simulink model "hydraulic_model"  (R2024a)
settings: Solver=ode23t  StartTime=0.0  StopTime=tEnd  FixedStep=1e-4  MaxStep=maxStep  RelTol=1e-2  AbsTol=1e-2
values from neighbouring files (symbols this model uses):
  boomHEArea = pi * (boomBoreDiameter/2)^2    (= 3117.24531052)    [init_model.m]
  boomREArea = pi * (boomBoreDiameter/2)^2 - pi*(boomRodDiameter/2)^2    (= 2410.38696347)    [init_model.m]
  swingDisplacement = 23.6    [init_model.m]
undefined symbols (not defined in the file or in its folder): ArmC, ArmR, AToTOrificeVector, BiPOrificeVector, BoomC, BoomR, boomValve, BToTOrificeVector, BucketC, BucketR, bucketValve, fluids, PToAOrificeVector, PToBOrificeVector, stickValve, SwingC, SwingR, swingValve, X, Y, Z
libraries: fl_lib x81, SimscapeFluids_lib x54, sm_lib x34, nesl_utility x29, spsFirstOrderFilterLib x4
(part 1 of 5)
settings Model: SimulationMode=accelerator  Creator=The MathWorks, Inc.  LastModifiedBy=jommsy
settings SolverCC: MaxConsecutiveMinStep=10  ZeroCrossAlgorithm=Adaptive  AlgebraicLoopSolver=TrustRegion  DecoupledContinuousIntegration=on  MinimalZcImpactIntegration=on
settings DataIOCC: SaveOutput=off  DSMLogging=off  OutputTimes=[0:0.02:20]
settings OptimizationCC: UseDivisionForNetSlopeComputation=UseDivisionForReciprocalsOfIntegersOnly  StateBitsets=on  DataBitsets=on
settings DebuggingCC: IgnoredZcDiagnostic=none  IntegerOverflowMsg=error  UnconnectedInputMsg=warning  UnconnectedOutputMsg=warning  UnconnectedLineMsg=warning  ArithmeticOperatorsInVariantConditions=warning
settings ModelReferenceCC: EnableRefExpFcnMdlSchedulingChecks=on
settings SFSimCC: MATLABDynamicMemAlloc=off  CustomCodeUndefinedFunction=UseInterfaceOnly
settings RTWCC: GPUComputeCapability=3.5
settings GRTTargetCC: UtilityFuncGeneration=Shared location
settings ExplorerConfigSet: SimMechanicsOpenEditorOnUpdate=off

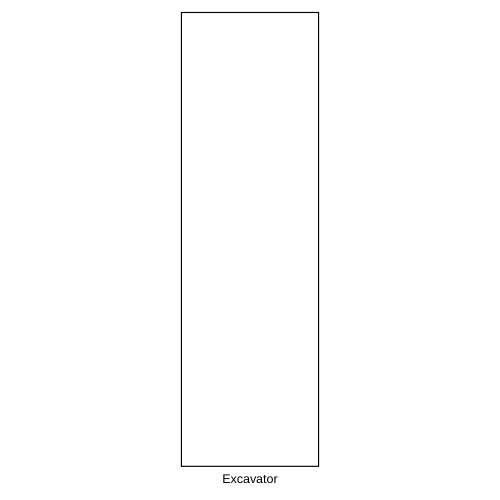
[thumbnail: Simulink's stored preview of the top-level diagram]
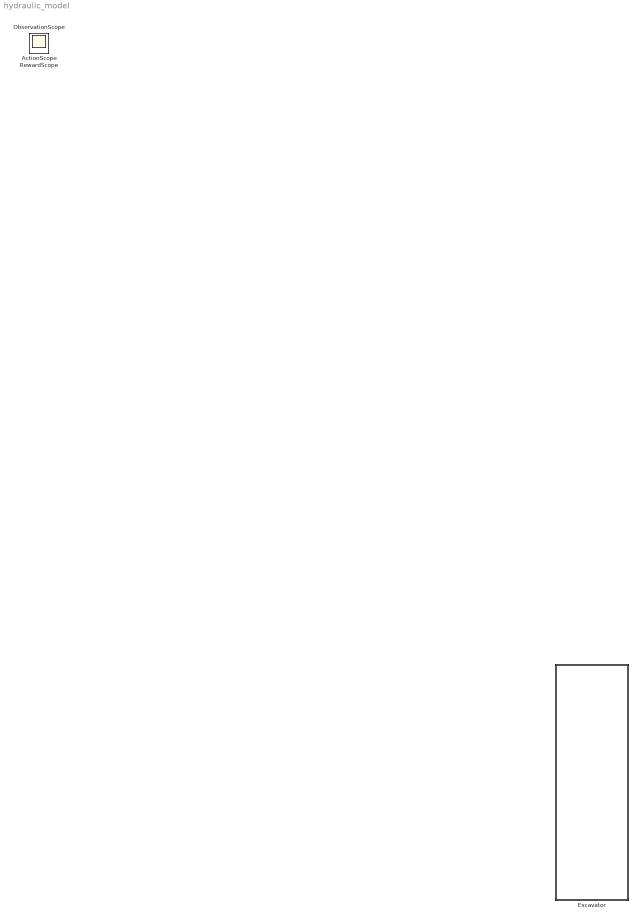
== system hydraulic_model ==
  Excavator : Subsystem
  ActionScope : Scope
  ObservationScope : Scope
  RewardScope : Scope

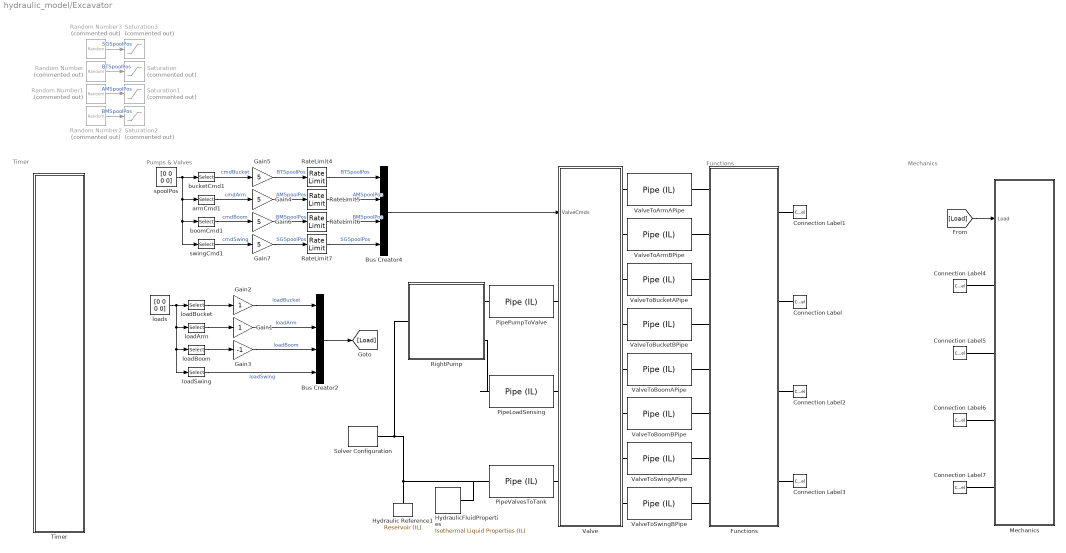
== system hydraulic_model/Excavator ==
  note: Functions
  note: Pumps & Valves
  note: Timer
  note: Mechanics
  Bus Creator2 : BusCreator  Inputs=4
  Bus Creator4 : BusCreator  Inputs=4
  Connection Label : ConnectionLabel  Label=ArmCyl
  Connection Label1 : ConnectionLabel  Label=BucketCyl
  Connection Label2 : ConnectionLabel  Label=BoomCyl
  Connection Label3 : ConnectionLabel  Label=SwingMotor
  Connection Label4 : ConnectionLabel  Label=ArmCyl
  Connection Label5 : ConnectionLabel  Label=BucketCyl
  Connection Label6 : ConnectionLabel  Label=BoomCyl
  Connection Label7 : ConnectionLabel  Label=SwingMotor
  Functions : Subsystem
      mask Display: image('Hydraulic_Actuators_All_IMAGE.png');
  Gain1 : Gain
  Gain2 : Gain
  Gain3 : Gain  Gain=-1
  Gain{4..7} (4 alike) : Gain  Gain=5
  Hydraulic Reference1 : fl_lib/Isothermal Liquid/Elements/Reservoir (IL)  reservoir_type=foundation.enum.constant_controlled.constant  pressure_spec=foundation.enum.pressure_spec.atmospheric  reservoir_pressure=0.101325 MPa
  HydraulicFluidProperties : fl_lib/Isothermal Liquid/Utilities/Isothermal Liquid Properties (IL)  rho_L_atm=870 kg/m^3  bulk_modulus_model=foundation.enum.bulk_modulus_model.const  beta_gain=6  beta_L_atm=1.45e9 Pa  nu_atm=46 mm^2/s  p_atm=0.101325 MPa  p_min=0.1 Pa  properties_range_check=simscape.enum.assert.action.error  air_fraction=0.005  polytropic_index=1.0  rho_g_atm=1.225 kg/m^3  air_dissolution_model=simscape.enum.onoff.off  p_crit=3 MPa
  Mechanics : Subsystem
      settings: PortSchema="{\"entries\":[{\"content\":{\"sides\":[{\"content\":{},\"type\":\"ConnectorPlacement.EquallySpacedRectSide\",\"uuid\":\"df542c6c-93e0-4cd8-a234-068f710ec41b\"},{\"content\":{\"side\":\"RIGHT\"},\"type\":\"ConnectorPlacement.EquallySpacedRectSide\",\"uuid\":\"8b36ef69-95bb-49de-9017-375655dff0aa\"},{\"content\":{\"connectorIds\":[\"In1\",\"LConn1\",\"LConn2\",\"LConn3\",\"LConn4\"],\"side\":\"TOP\"},\"type\":\"ConnectorPlacement.EquallySpacedRectSide\",\"uuid\":\"d3e749b5-c6b1-4a0f-a6f8-f63c6bfd6ba8\"}]},\"type\":\"ConnectorPlacement.EquallySpacedConnector\",\"uuid\":\"9d57a862-0266-4ba5-b197-b3f576208194\"}],\"packageUris\":[\"http://schema.mathworks.com/mf0/Connector/R2020b\"],\"version\":\"1.0\"}"
      mask Display: image('Excavator_Cylinder_CalcForce_IMAGE.png', [0,0,0,0,80,80]);
  PipeLoadSensing : fl_lib/Isothermal Liquid/Elements/Pipe (IL)  length=pipeLength mm  area=pipeCrossSectArea mm^2  Dh=pipeHydraulicDiam mm  length_add=1 m  roughness=15e-6 m  Re_lam=2000  Re_tur=4000  shape_factor=64  dynamic_compressibility=simscape.enum.onoff.off  inertia=simscape.enum.onoff.off  p0=0.101325 MPa  mdot0=0 kg/s
      settings: InternalSimscapePortConfiguration="{\"Bottom\":[],\"Left\":[{\"id\":\"A\",\"label\":\"A\",\"type\":\"foundation.isothermal_liquid.isothermal_liquid\"}],\"Right\":[{\"id\":\"B\",\"label\":\"B\",\"type\":\"foundation.isothermal_liquid.isothermal_liquid\"}],\"Top\":[]}"
  PipePumpToValve : fl_lib/Isothermal Liquid/Elements/Pipe (IL)  length=pipeLength mm  area=pipeCrossSectArea mm^2  Dh=pipeHydraulicDiam mm  length_add=1 m  roughness=15e-6 m  Re_lam=2000  Re_tur=4000  shape_factor=64  dynamic_compressibility=simscape.enum.onoff.off  inertia=simscape.enum.onoff.off  p0=0.101325 MPa  mdot0=0 kg/s
      settings: InternalSimscapePortConfiguration="{\"Bottom\":[],\"Left\":[{\"id\":\"A\",\"label\":\"A\",\"type\":\"foundation.isothermal_liquid.isothermal_liquid\"}],\"Right\":[{\"id\":\"B\",\"label\":\"B\",\"type\":\"foundation.isothermal_liquid.isothermal_liquid\"}],\"Top\":[]}"
  PipeValvesToTank : fl_lib/Isothermal Liquid/Elements/Pipe (IL)  length=pipeLength mm  area=pipeCrossSectArea mm^2  Dh=pipeHydraulicDiam mm  length_add=1 m  roughness=15e-6 m  Re_lam=2000  Re_tur=4000  shape_factor=64  dynamic_compressibility=simscape.enum.onoff.off  inertia=simscape.enum.onoff.off  p0=0.101325 MPa  mdot0=0 kg/s
      settings: InternalSimscapePortConfiguration="{\"Bottom\":[],\"Left\":[{\"id\":\"A\",\"label\":\"A\",\"type\":\"foundation.isothermal_liquid.isothermal_liquid\"}],\"Right\":[{\"id\":\"B\",\"label\":\"B\",\"type\":\"foundation.isothermal_liquid.isothermal_liquid\"}],\"Top\":[]}"
  Random Number : RandomNumber  Commented=on  Variance=0.3  SampleTime=0.02
  Random Number1 : RandomNumber  Commented=on  Variance=0.3  Seed=1000  SampleTime=0.02
  Random Number2 : RandomNumber  Commented=on  Variance=0.3  Seed=20  SampleTime=0.02
  Random Number3 : RandomNumber  Commented=on  Variance=0.3  Seed=800  SampleTime=0.02
  RateLimit{4..7} (4 alike) : RateLimiter  RisingSlewLimit=7.5  FallingSlewLimit=-7.5  SampleTimeMode=inherited
  RightPump : Subsystem
      mask Display: image('Hydraulic_Pump_IMAGE.png');
  Saturation{,1..3} (4 alike) : Saturate  Commented=on  UpperLimit=1  LowerLimit=-1
  Solver Configuration : nesl_utility/Solver Configuration  PhysicalDomain=network_engine_domain  SubClassName=solver  LeftPortType=input  RightPortType=generic  Tones=[]  Harmonics=[]  SimulateNoise=off  Profile=off  UseLocalSampling=off  EnableSwitchedLinearOptims=on  FrequencyDomain=off  UseCCode=off  RelTol=0.001  AbsTol=0.001  MinStep=1e-09  ToWorkspace=off  RevertToSquareIcSolve=off  NumHomotopyIterations=100  PhasorMode=off  PhasorModeNumHarmonics=1  ConsistencySolver=NEWTON_XTOL_AFTER_FTOL  IndexReductionMethod=DerivativeReplacement  DoDC=off  ResidualTolerance=1e-09  ConsistencyTolSource=GLOBAL  ConsistencyAbsTol=0.001  ConsistencyRelTol=0.001  ConsistencyTolFactor=1  UseLocalSolver=off  LocalSolverChoice=NE_BACKWARD_EULER_ADVANCER  ResolveIndetEquations=on  FunctionEvalNumThread=1  LocalSolverSampleTime=0.001  DoFixedCost=off  MaxNonlinIter=3  MaxModeIter=2  ComputeImpulses=off  ImpulseIterations=2  LinearAlgebra=auto  LinearAlgebraNumThread=0  EquationFormulation=NE_TIME_EF  DelaysMemoryBudget=1024  AutomaticFiltering=on  FilteringTimeConstant=0.01  PartitionStorageMethod=AS_NEEDED  PartitionMemoryBudget=1024  PartitionMethod=ROBUST  MultibodyUseLocalSolver=off  MultibodyLocalSolverChoice=ODE1  MultibodyLocalSolverSampleTime=0.001
  Timer : Subsystem
      mask Display: image('Timer.png', [0,0,0,0,100,50]);
  Valve : Subsystem
      mask Display: image('Valve_Block_All_IMAGE.png');
  ValveToArmAPipe : fl_lib/Isothermal Liquid/Elements/Pipe (IL)  length=pipeLength mm  area=pipeCrossSectArea mm^2  Dh=pipeHydraulicDiam mm  length_add=1 m  roughness=15e-6 m  Re_lam=2000  Re_tur=4000  shape_factor=64  dynamic_compressibility=simscape.enum.onoff.off  inertia=simscape.enum.onoff.off  p0=0.101325 MPa  mdot0=0 kg/s
      settings: InternalSimscapePortConfiguration="{\"Bottom\":[],\"Left\":[{\"id\":\"A\",\"label\":\"A\",\"type\":\"foundation.isothermal_liquid.isothermal_liquid\"}],\"Right\":[{\"id\":\"B\",\"label\":\"B\",\"type\":\"foundation.isothermal_liquid.isothermal_liquid\"}],\"Top\":[]}"
  ValveToArmBPipe : fl_lib/Isothermal Liquid/Elements/Pipe (IL)  length=pipeLength mm  area=pipeCrossSectArea mm^2  Dh=pipeHydraulicDiam mm  length_add=1 m  roughness=15e-6 m  Re_lam=2000  Re_tur=4000  shape_factor=64  dynamic_compressibility=simscape.enum.onoff.off  inertia=simscape.enum.onoff.off  p0=0.101325 MPa  mdot0=0 kg/s
      settings: InternalSimscapePortConfiguration="{\"Bottom\":[],\"Left\":[{\"id\":\"A\",\"label\":\"A\",\"type\":\"foundation.isothermal_liquid.isothermal_liquid\"}],\"Right\":[{\"id\":\"B\",\"label\":\"B\",\"type\":\"foundation.isothermal_liquid.isothermal_liquid\"}],\"Top\":[]}"
  ValveToBoomAPipe : fl_lib/Isothermal Liquid/Elements/Pipe (IL)  length=pipeLength mm  area=pipeCrossSectArea mm^2  Dh=pipeHydraulicDiam mm  length_add=1 m  roughness=15e-6 m  Re_lam=2000  Re_tur=4000  shape_factor=64  dynamic_compressibility=simscape.enum.onoff.off  inertia=simscape.enum.onoff.off  p0=0.101325 MPa  mdot0=0 kg/s
      settings: InternalSimscapePortConfiguration="{\"Bottom\":[],\"Left\":[{\"id\":\"A\",\"label\":\"A\",\"type\":\"foundation.isothermal_liquid.isothermal_liquid\"}],\"Right\":[{\"id\":\"B\",\"label\":\"B\",\"type\":\"foundation.isothermal_liquid.isothermal_liquid\"}],\"Top\":[]}"
  ValveToBoomBPipe : fl_lib/Isothermal Liquid/Elements/Pipe (IL)  length=pipeLength mm  area=pipeCrossSectArea mm^2  Dh=pipeHydraulicDiam mm  length_add=1 m  roughness=15e-6 m  Re_lam=2000  Re_tur=4000  shape_factor=64  dynamic_compressibility=simscape.enum.onoff.off  inertia=simscape.enum.onoff.off  p0=0.101325 MPa  mdot0=0 kg/s
      settings: InternalSimscapePortConfiguration="{\"Bottom\":[],\"Left\":[{\"id\":\"A\",\"label\":\"A\",\"type\":\"foundation.isothermal_liquid.isothermal_liquid\"}],\"Right\":[{\"id\":\"B\",\"label\":\"B\",\"type\":\"foundation.isothermal_liquid.isothermal_liquid\"}],\"Top\":[]}"
  ValveToBucketAPipe : fl_lib/Isothermal Liquid/Elements/Pipe (IL)  length=pipeLength mm  area=pipeCrossSectArea mm^2  Dh=pipeHydraulicDiam mm  length_add=1 m  roughness=15e-6 m  Re_lam=2000  Re_tur=4000  shape_factor=64  dynamic_compressibility=simscape.enum.onoff.off  inertia=simscape.enum.onoff.off  p0=0.101325 MPa  mdot0=0 kg/s
      settings: InternalSimscapePortConfiguration="{\"Bottom\":[],\"Left\":[{\"id\":\"A\",\"label\":\"A\",\"type\":\"foundation.isothermal_liquid.isothermal_liquid\"}],\"Right\":[{\"id\":\"B\",\"label\":\"B\",\"type\":\"foundation.isothermal_liquid.isothermal_liquid\"}],\"Top\":[]}"
  ValveToBucketBPipe : fl_lib/Isothermal Liquid/Elements/Pipe (IL)  length=pipeLength mm  area=pipeCrossSectArea mm^2  Dh=pipeHydraulicDiam mm  length_add=1 m  roughness=15e-6 m  Re_lam=2000  Re_tur=4000  shape_factor=64  dynamic_compressibility=simscape.enum.onoff.off  inertia=simscape.enum.onoff.off  p0=0.101325 MPa  mdot0=0 kg/s
      settings: InternalSimscapePortConfiguration="{\"Bottom\":[],\"Left\":[{\"id\":\"A\",\"label\":\"A\",\"type\":\"foundation.isothermal_liquid.isothermal_liquid\"}],\"Right\":[{\"id\":\"B\",\"label\":\"B\",\"type\":\"foundation.isothermal_liquid.isothermal_liquid\"}],\"Top\":[]}"
  ValveToSwingAPipe : fl_lib/Isothermal Liquid/Elements/Pipe (IL)  length=pipeLength mm  area=pipeCrossSectArea mm^2  Dh=pipeHydraulicDiam mm  length_add=1 m  roughness=15e-6 m  Re_lam=2000  Re_tur=4000  shape_factor=64  dynamic_compressibility=simscape.enum.onoff.off  inertia=simscape.enum.onoff.off  p0=0.101325 MPa  mdot0=0 kg/s
      settings: InternalSimscapePortConfiguration="{\"Bottom\":[],\"Left\":[{\"id\":\"A\",\"label\":\"A\",\"type\":\"foundation.isothermal_liquid.isothermal_liquid\"}],\"Right\":[{\"id\":\"B\",\"label\":\"B\",\"type\":\"foundation.isothermal_liquid.isothermal_liquid\"}],\"Top\":[]}"
  ValveToSwingBPipe : fl_lib/Isothermal Liquid/Elements/Pipe (IL)  length=pipeLength mm  area=pipeCrossSectArea mm^2  Dh=pipeHydraulicDiam mm  length_add=1 m  roughness=15e-6 m  Re_lam=2000  Re_tur=4000  shape_factor=64  dynamic_compressibility=simscape.enum.onoff.off  inertia=simscape.enum.onoff.off  p0=0.101325 MPa  mdot0=0 kg/s
      settings: InternalSimscapePortConfiguration="{\"Bottom\":[],\"Left\":[{\"id\":\"A\",\"label\":\"A\",\"type\":\"foundation.isothermal_liquid.isothermal_liquid\"}],\"Right\":[{\"id\":\"B\",\"label\":\"B\",\"type\":\"foundation.isothermal_liquid.isothermal_liquid\"}],\"Top\":[]}"
  armCmd1 : Selector  InputPortWidth=4  IndexOptions=Index vector (dialog)  Indices=3  OutputSizes=1
  boomCmd1 : Selector  InputPortWidth=4  IndexOptions=Index vector (dialog)  Indices=2  OutputSizes=1
  bucketCmd1 : Selector  InputPortWidth=4  IndexOptions=Index vector (dialog)  Indices=4  OutputSizes=1
  loadArm : Selector  InputPortWidth=4  IndexOptions=Index vector (dialog)  Indices=3  OutputSizes=1
  loadBoom : Selector  InputPortWidth=4  IndexOptions=Index vector (dialog)  Indices=2  OutputSizes=1
  loadBucket : Selector  InputPortWidth=4  IndexOptions=Index vector (dialog)  Indices=4  OutputSizes=1
  loadSwing : Selector  InputPortWidth=4  IndexOptions=Index vector (dialog)  Indices=1  OutputSizes=1
  loads : Constant  Value=[0 0 0 0]  SampleTime=0.02
  spoolPos : Constant  Value=[0 0 0 0]  SampleTime=0.02
  swingCmd1 : Selector  InputPortWidth=4  IndexOptions=Index vector (dialog)  Indices=1  OutputSizes=1
  wires:
  [Load] -> Mechanics/1(Load)
  Bus Creator2/1 -> [Load]
  Bus Creator4/1 -> Valve/1(ValveCmds)
  Gain4/1 -> RateLimit5/1  "AMSpoolPos"
  RateLimit5/1 -> Bus Creator4/2  "AMSpoolPos"
  RateLimit4/1 -> Bus Creator4/1  "BTSpoolPos"
  Gain5/1 -> RateLimit4/1  "BTSpoolPos"
  armCmd1/1 -> Gain4/1  "cmdArm"
  swingCmd1/1 -> Gain7/1  "cmdSwing"
  RateLimit6/1 -> Bus Creator4/3  "BMSpoolPos"
  bucketCmd1/1 -> Gain5/1  "cmdBucket"
  boomCmd1/1 -> Gain6/1  "cmdBoom"
  RateLimit7/1 -> Bus Creator4/4  "SGSpoolPos"
  Gain7/1 -> RateLimit7/1  "SGSpoolPos"
  Gain6/1 -> RateLimit6/1  "BMSpoolPos"
  Gain2/1 -> Bus Creator2/1  "loadBucket"
  Gain1/1 -> Bus Creator2/2  "loadArm"
  Gain3/1 -> Bus Creator2/3  "loadBoom"
  loadSwing/1 -> Bus Creator2/4  "loadSwing"
  loadBucket/1 -> Gain2/1
  loadArm/1 -> Gain1/1
  loads/1 -> loadSwing/1, loadBoom/1, loadArm/1, loadBucket/1
  loadBoom/1 -> Gain3/1
  spoolPos/1 -> bucketCmd1/1, armCmd1/1, boomCmd1/1, swingCmd1/1
  Random Number2/1 -> Saturation2/1  "BMSpoolPos"
  Random Number1/1 -> Saturation1/1  "AMSpoolPos"
  Random Number3/1 -> Saturation3/1  "SGSpoolPos"
  Random Number/1 -> Saturation/1  "BTSpoolPos"
  connections:
  Hydraulic Reference1/LConn1 -- HydraulicFluidProperties/RConn1 -- PipeValvesToTank/RConn1 -- Solver Configuration/RConn1 -- RightPump/LConn1
  ValveToArmBPipe/RConn1 -- Functions/LConn2
  Valve/RConn8 -- ValveToSwingBPipe/LConn1
  ValveToBucketBPipe/RConn1 -- Functions/LConn4
  Valve/RConn5 -- ValveToBoomAPipe/LConn1
  ValveToArmAPipe/RConn1 -- Functions/LConn1
  ValveToSwingBPipe/RConn1 -- Functions/LConn8
  ValveToBucketAPipe/RConn1 -- Functions/LConn3
  Valve/RConn7 -- ValveToSwingAPipe/LConn1
  ValveToBoomAPipe/RConn1 -- Functions/LConn5
  Valve/RConn4 -- ValveToBucketBPipe/LConn1
  Valve/RConn1 -- ValveToArmAPipe/LConn1
  ValveToBoomBPipe/RConn1 -- Functions/LConn6
  ValveToSwingAPipe/RConn1 -- Functions/LConn7
  Valve/RConn6 -- ValveToBoomBPipe/LConn1
  Valve/RConn3 -- ValveToBucketAPipe/LConn1
  Valve/RConn2 -- ValveToArmBPipe/LConn1
  Valve/LConn3 -- PipeValvesToTank/LConn1
  Valve/LConn1 -- PipePumpToValve/RConn1
  RightPump/RConn1 -- PipePumpToValve/LConn1
  PipeLoadSensing/RConn1 -- Valve/LConn2
  PipeLoadSensing/LConn1 -- RightPump/RConn2
  Connection Label7/LConn1 -- Mechanics/LConn4
  Connection Label4/LConn1 -- Mechanics/LConn1
  Connection Label5/LConn1 -- Mechanics/LConn2
  Connection Label6/LConn1 -- Mechanics/LConn3
  Connection Label1/LConn1 -- Functions/RConn1
  Connection Label/LConn1 -- Functions/RConn2
  Connection Label2/LConn1 -- Functions/RConn3
  Connection Label3/LConn1 -- Functions/RConn4

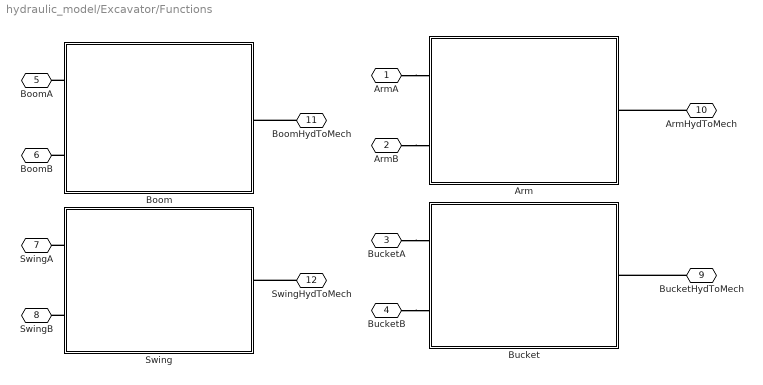
== system hydraulic_model/Excavator/Functions ==
  Arm : Subsystem
      mask Display: image('Actuator_1Cyl_IMAGE.png');
  Boom : Subsystem
      mask Display: image('Actuator_1Cyl_IMAGE.png');
  Bucket : Subsystem
      mask Display: image('Actuator_1Cyl_IMAGE.png');
  Swing : Subsystem
      mask Display: image('Actuator_1Motor_IMAGE.png');
  ArmA : PMIOPort  Side=Left
  ArmB : PMIOPort  Port=2  Side=Left
  BucketA : PMIOPort  Port=3  Side=Left
  BucketB : PMIOPort  Port=4  Side=Left
  BoomA : PMIOPort  Port=5  Side=Left
  BoomB : PMIOPort  Port=6  Side=Left
  SwingA : PMIOPort  Port=7  Side=Left
  SwingB : PMIOPort  Port=8  Side=Left
  BucketHydToMech : PMIOPort  Port=9  Side=Right
  ArmHydToMech : PMIOPort  Port=10  Side=Right
  BoomHydToMech : PMIOPort  Port=11  Side=Right
  SwingHydToMech : PMIOPort  Port=12  Side=Right
  connections:
  Swing/LConn2 -- SwingB/RConn1
  BucketA/RConn1 -- Bucket/LConn1
  ArmA/RConn1 -- Arm/LConn1
  BucketB/RConn1 -- Bucket/LConn2
  ArmB/RConn1 -- Arm/LConn2
  Boom/LConn2 -- BoomB/RConn1
  Boom/LConn1 -- BoomA/RConn1
  Swing/LConn1 -- SwingA/RConn1
  BoomHydToMech/RConn1 -- Boom/RConn1
  ArmHydToMech/RConn1 -- Arm/RConn1
  SwingHydToMech/RConn1 -- Swing/RConn1
  BucketHydToMech/RConn1 -- Bucket/RConn1

== system hydraulic_model/Excavator/Mechanics ==
  Load : Inport
  Arm : Subsystem
      mask Display: image('Excavator_Cylinder_Actuate_IMAGE.png');
  Boom : Subsystem
      mask Display: image('Excavator_Cylinder_Actuate_IMAGE.png');
  Bucket : Subsystem
      mask Display: image('Excavator_Cylinder_Actuate_IMAGE.png');
  Cabin : Subsystem
      mask Display: image('Excavator_Revolute_Actuate_IMAGE.png');
  Load to Cylinders : Subsystem
  Mechanism Configuration : sm_lib/Utilities/Mechanism Configuration  UniformGravity=Constant  GravityVector=[0 0 -9.80665]  GravityVectorUnits=m/s^2  LinearizationDelta=0.001  JointModeTransitionNonlinearIterations=2
  World Frame : sm_lib/Frames and Transforms/World Frame
  ArmHyd : PMIOPort  Side=Left
  BucketHyd : PMIOPort  Port=2  Side=Left
  BoomHyd : PMIOPort  Port=3  Side=Left
  SwingHyd : PMIOPort  Port=4  Side=Left
  wires:
  Load/1 -> Load to Cylinders/1(Loads1)
  connections:
  Mechanism Configuration/RConn1 -- Cabin/LConn1 -- Boom/RConn1 -- Arm/RConn1 -- Bucket/RConn1 -- World Frame/RConn1
  BoomHyd/RConn1 -- Boom/RConn2
  ArmHyd/RConn1 -- Arm/RConn2
  BucketHyd/RConn1 -- Bucket/RConn2
  Bucket/LConn1 -- Load to Cylinders/RConn1
  SwingHyd/RConn1 -- Cabin/LConn2
  Arm/LConn1 -- Load to Cylinders/RConn2
  Boom/LConn1 -- Load to Cylinders/RConn3
  Load to Cylinders/RConn4 -- Cabin/RConn1

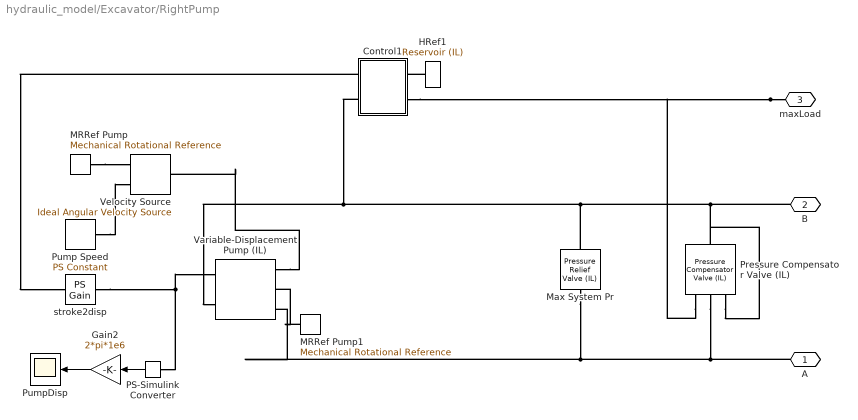
== system hydraulic_model/Excavator/RightPump ==
  Control1 : Subsystem  Tag=PublishSubsystem  mask(Load-sensing Pump Control Unit){servo_cyl_stroke=0.009, pump_stroke=0.009, servo_cyl_area=6e-4, servo_cyl_preload=1.4, servo_cyl_max_force=62, area_X=2e-4, area_Y=2e-4, press_diff=17e5, press_max=245e5, delta_p=1.5e5, valve_max_area=0.14, spool_stroke=5, x0_PA=-2.5, x0_AT=2.5}
      mask prompts: servo_cyl_stroke "Servo-cylinder stroke (m)"; pump_stroke "Pump control member stroke (m)"; servo_cyl_area "Servo-cylinder area (m^2)"; servo_cyl_preload "Servo-cylinder preload force (N)"; servo_cyl_max_force "Servo-cylinder maximum force (N)"; area_X "Spool face area X (m^2)"; area_Y "Spool face area Y (m^2)"; press_diff "Pressure differential (Pa)"; press_max "Maximum pump pressure (Pa)"; delta_p "Pressure differential delta (Pa)"; valve_max_area "Valve orifice maximum area (cm^2)"; spool_stroke "Spool stroke (mm)"; x0_PA "Orifice P-A initial opening (mm)"; x0_AT "Orifice A-T initial opening (mm)"
      mask help:
      | The unit is intended to maintain a preset pressure differential between ports P and A by changing the pump displacement through its control member C. The unit is also equipped with the pressure limiter which does not allow pump output pressure to
      | exceed preset value.
  Gain2 : Gain  Gain=2*pi*1e6
  HRef1 : fl_lib/Isothermal Liquid/Elements/Reservoir (IL)  Tag=Factory Generic  reservoir_type=foundation.enum.constant_controlled.constant  pressure_spec=foundation.enum.pressure_spec.atmospheric  reservoir_pressure=0.101325 MPa
  MRRef Pump : fl_lib/Mechanical/Rotational Elements/Mechanical Rotational Reference  Tag=Factory Generic
  MRRef Pump1 : fl_lib/Mechanical/Rotational Elements/Mechanical Rotational Reference  Tag=Factory Generic
  Max System Pr : SimscapeFluids_lib/Isothermal Liquid/Valves & Orifices/Pressure Control Valves/Pressure Relief Valve (IL)  set_pressure_spec=foundation.enum.constant_controlled.constant  opening_spec=fluids.isothermal_liquid.valves_orifices.enum.PressureOpeningSpec.Linear  pressure_spec=fluids.isothermal_liquid.valves_orifices.enum.pressure_control_spec.dp  p_set_gauge=0.1 MPa  p_set_differential=225 bar  p_range=5 bar  area_max=1200 mm^2  area_leak=0.001 mm^2  p_diff_TLU=[0.2 : 0.2 : 1.2] MPa  p_gauge_TLU=[0.2 : 0.2 : 1.2] MPa  valve_area_TLU=[1e-10, 2e-06, 4e-06, 6e-06, 8e-06, 1e-05] m^2  vol_flow_TLU=[1e-09, 3.6e-05, 8.9e-05, .00015, .00023, .00031] m^3/s  area=inf m^2  Cd=0.64  Re_c=150  smoothing_factor=0.01  pressure_recovery=true  opening_dynamics=false  tau=0.1 s  enable_faults=simscape.enum.onoff.off  fault_type=fluids.enum.FaultOpening.Closed
      settings: InternalSimscapePortConfiguration="{\"Bottom\":[],\"Left\":[{\"id\":\"A\",\"label\":\"A\",\"type\":\"foundation.isothermal_liquid.isothermal_liquid\"}],\"Right\":[{\"id\":\"B\",\"label\":\"B\",\"type\":\"foundation.isothermal_liquid.isothermal_liquid\"}],\"Top\":[]}"
  PS-Simulink Converter : nesl_utility/PS-Simulink Converter  PhysicalDomain=network_engine_domain  SubClassName=ps_output  LeftPortType=input  RightPortType=output  PseudoPeriodic=off  Frequencies=[]  VectorFormat=inherit  Unit=inherit  AffineConversion=off
  Pressure Compensator Valve (IL) : SimscapeFluids_lib/Isothermal Liquid/Valves & Orifices/Pressure Control Valves/Pressure Compensator Valve (IL)  valve_spec=fluids.isothermal_liquid.valves_orifices.enum.closed_open.closed  set_pressure_spec=foundation.enum.constant_controlled.constant  opening_spec=fluids.isothermal_liquid.valves_orifices.enum.opening_spec.linear  p_set_differential=21 bar  p_range=0.5 bar  area_max=100 mm^2  area_leak=1e-4 mm^2  p_diff_reducing_TLU=[0.2 : 0.2 : 1.2] MPa  valve_area_reducing_TLU=[1e-05, 8e-06, 6e-06, 4e-06, 2e-06, 1e-10] m^2  p_diff_relief_TLU=[0.2 : 0.2 : 1.2] MPa  valve_area_relief_TLU=[1e-10, 2e-06, 4e-06, 6e-06, 8e-06, 1e-05] m^2  area=inf m^2  Cd=0.64  Re_c=150  smoothing_factor=0.01  pressure_recovery=false  opening_dynamics=false  tau=0.1 s  enable_faults=simscape.enum.onoff.off  fault_type=fluids.enum.FaultOpening.Closed  faulted_specify=off  faulted_priority=High  faulted=0
      settings: InternalSimscapePortConfiguration="{\"Bottom\":[],\"Left\":[{\"id\":\"A\",\"label\":\"A\",\"type\":\"foundation.isothermal_liquid.isothermal_liquid\"}],\"Right\":[{\"id\":\"X\",\"label\":\"X\",\"type\":\"foundation.isothermal_liquid.isothermal_liquid\"},{\"id\":\"B\",\"label\":\"B\",\"type\":\"foundation.isothermal_liquid.isothermal_liquid\"},{\"id\":\"Y\",\"label\":\"Y\",\"type\":\"foundation.isothermal_liquid.isothermal_liquid\"}],\"Top\":[]}"
  Pump Speed : fl_lib/Physical Signals/Sources/PS Constant  constant=pumpSpeed rpm
  PumpDisp : Scope
  Variable-Displacement Pump (IL) : SimscapeFluids_lib/Isothermal Liquid/Pumps & Motors/Variable-Displacement Pump (IL)  leakage_friction_spec=fluids.isothermal_liquid.pumps_motors.enum.pump_motor_loss_spec.analytical  displacement_nominal=30 cm^3/rev  omega_nominal=2000 rpm  p_nominal=24.5 MPa  vol_eff_nominal=0.92  mech_eff_nominal=0.88  no_load_torque=0 N*m  p_diff_eff_TLU=[.1, 1, 2] MPa  omega_eff_TLU=[250, 500, 1000, 2000, 3000, 4000] rpm  displacement_eff_TLU=[-30, -19, 19, 30] cm^3/rev  vol_eff_TLU=repmat([.816, .908, .954, .977, .981, .984; .325, .663, .831, .916, .925, .946; .137, .568, .78, .892, .893, .91], 1, 1, 4)  mech_eff_TLU=repmat([.996, .996, .996, .996, .996, .996; .988, .989, .989, .989, .989, .99; .981, .981, .982, .982, .983, .984], 1, 1, 4)  p_diff_loss_TLU=[.1, 1, 2] MPa  omega_loss_TLU=[250, 500, 1000, 2000, 3000, 4000] rpm  displacement_loss_TLU=[-30, -19, 19, 30] cm^3/rev  vol_loss_TLU=repmat(1e-3 * [.023, .023, .023, .023, .0285, .032; .0844, .0842, .0845, .084, .1125, .108; .1079, .108, .11, .108, .1605, .18], 1, 1, 4) m^3/s  mech_loss_TLU=repmat([.002, .002, .002, .002, .002, .002; .0607, .0556, .0556, .0556, .0556, .0505; .1937, .1937, .1833, .1833, .1729, .1626], 1, 1, 4) N*m  vol_eff_min=1e-3  vol_eff_max=1  mech_eff_min=1e-3  mech_eff_max=1  pressure_threshold=1e-3 MPa  omega_threshold=100 rpm  displacement_threshold=0.1 cm^3/rev  supplied_range_check=simscape.enum.assert.action.none  pump_mode_check=simscape.enum.assert.action.none  pressure_check=simscape.enum.assert.action.none  p_min_valid=0.101325 MPa
      settings: InternalSimscapePortConfiguration="{\"Bottom\":[{\"id\":\"A\",\"label\":\"A\",\"type\":\"foundation.isothermal_liquid.isothermal_liquid\"}],\"Left\":[{\"id\":\"D\",\"label\":\"D\",\"type\":\"input\"}],\"Right\":[{\"id\":\"R\",\"label\":\"R\",\"type\":\"foundation.mechanical.rotational.rotational\"},{\"id\":\"C\",\"label\":\"C\",\"type\":\"foundation.mechanical.rotational.rotational\"}],\"Top\":[{\"id\":\"B\",\"label\":\"B\",\"type\":\"foundation.isothermal_liquid.isothermal_liquid\"}]}"
  Velocity Source : fl_lib/Mechanical/Mechanical Sources/Ideal Angular Velocity Source  Tag=Factory Generic
  stroke2disp : fl_lib/Physical Signals/Functions/PS Gain  gain=(4.8e-06)/(0.009) m^2/rad
  A : PMIOPort  Side=Left
  B : PMIOPort  Port=2  Side=Right
  maxLoad : PMIOPort  Port=3  Side=Right
  wires:
  PS-Simulink Converter/1 -> Gain2/1
  Gain2/1 -> PumpDisp/1
  connections:
  MRRef Pump/LConn1 -- Velocity Source/RConn2
  Pump Speed/RConn1 -- Velocity Source/RConn1
  Variable-Displacement Pump (IL)/RConn1 -- Velocity Source/LConn1
  HRef1/LConn1 -- Control1/RConn1
  B/RConn1 -- Pressure Compensator Valve (IL)/RConn1 -- Pressure Compensator Valve (IL)/LConn1 -- Max System Pr/LConn1 -- Control1/LConn2 -- Variable-Displacement Pump (IL)/LConn2
  maxLoad/RConn1 -- Control1/RConn2 -- Pressure Compensator Valve (IL)/RConn3
  Control1/LConn1 -- stroke2disp/LConn1
  A/RConn1 -- Pressure Compensator Valve (IL)/RConn2 -- Variable-Displacement Pump (IL)/RConn3 -- Max System Pr/RConn1
  MRRef Pump1/LConn1 -- Variable-Displacement Pump (IL)/RConn2
  stroke2disp/RConn1 -- PS-Simulink Converter/LConn1 -- Variable-Displacement Pump (IL)/LConn1

== system hydraulic_model/Excavator/Timer ==
  Assertion1 : Assertion  AssertionFailFcn=|  StopWhenAssertionFail=off
      | set_param('hydraulic_model', 'SimulationCommand', 'pause');
      | Tmp = get_param('hydraulic_model', 'SimulationTime');
      | set_param('hydraulic_model/Excavator/Timer/Tmp', 'Value', num2str(Tmp));
  Clock : Clock
  MATLAB Function : MATLAB Function  TreatAsAtomicUnit=on
  Relational Operator : RelationalOperator  OutDataTypeStr=boolean  RndMeth=Simplest  InputSameDT=off
  Tmp : Constant  Value=0
  Ts : Constant  Value=0
  wires:
  Relational Operator/1 -> Assertion1/1
  Tmp/1 -> MATLAB Function/2(Tmp)
  MATLAB Function/1(time_differ) -> Relational Operator/2
  Clock/1 -> MATLAB Function/1(current_time)
  Ts/1 -> Relational Operator/1
